simulink model "Problem1"  (R2020b)
settings: Solver=VariableStepAuto  StartTime=0.0  StopTime=100  RelTol=1e-3
model workspace (MAT data in the model file):
  b = 50
  k1 = 50
  k12 = 10000
  m1 = 100
  m2 = 100
settings Model: OrderedModelArguments=off  Creator=Acer  LastModifiedBy=Acer

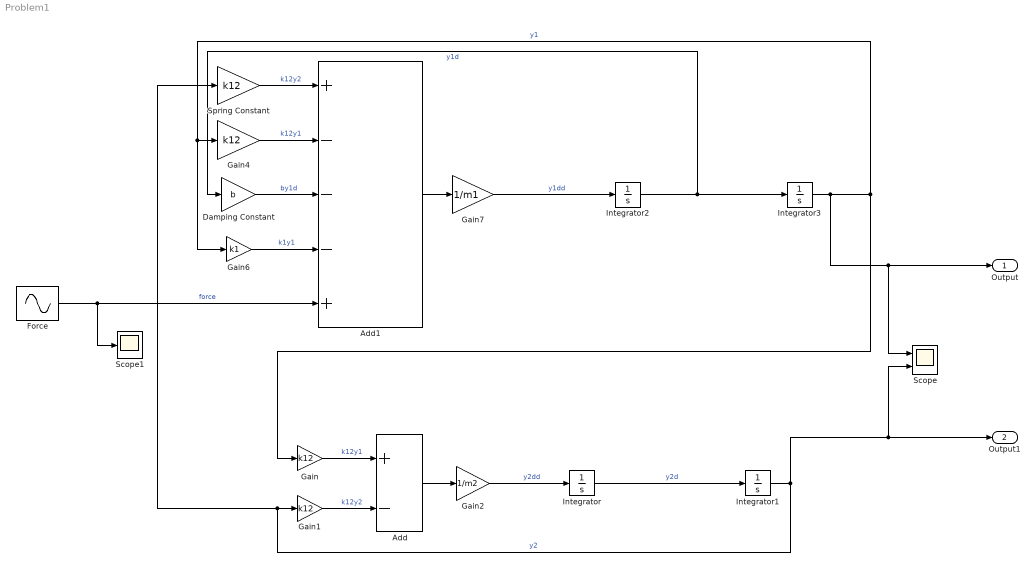
== system Problem1 ==
  Add : Sum  Inputs=+-
  Add1 : Sum  Inputs=+---+
  Damping Constant : Gain  Gain=b
  Force : Sin  Amplitude=2  Frequency=10  SampleTime=0.001
  Gain : Gain  Gain=k12
  Gain1 : Gain  Gain=k12
  Gain2 : Gain  Gain=1/m2
  Gain4 : Gain  Gain=k12
  Gain6 : Gain  Gain=k1
  Gain7 : Gain  Gain=1/m1
  Integrator{,1..3} (4 alike) : Integrator
  Scope : Scope  NumInputPorts=2
  Scope1 : Scope
  Spring Constant : Gain  Gain=k12
  Output : Outport
  Output1 : Outport  Port=2
  wires:
  Integrator/1 -> Integrator1/1  "y2d"
  Integrator1/1 -> Spring Constant/1, Gain1/1, Output1/1, Scope/2  "y2"
  Gain2/1 -> Integrator/1  "y2dd"
  Integrator2/1 -> Damping Constant/1, Integrator3/1  "y1d"
  Integrator3/1 -> Gain/1, Gain4/1, Gain6/1, Scope/1, Output/1  "y1"
  Gain7/1 -> Integrator2/1  "y1dd"
  Gain/1 -> Add/1  "k12y1"
  Gain1/1 -> Add/2  "k12y2"
  Add/1 -> Gain2/1
  Spring Constant/1 -> Add1/1  "k12y2"
  Gain4/1 -> Add1/2  "k12y1"
  Damping Constant/1 -> Add1/3  "by1d"
  Gain6/1 -> Add1/4  "k1y1"
  Add1/1 -> Gain7/1
  Force/1 -> Add1/5, Scope1/1  "force"
